simulink model "PID_Controller"  (R2020b)
settings: Solver=VariableStepAuto  StartTime=0.0  StopTime=1  FixedStep=Ts  RelTol=1e-3
model workspace (MAT data in the model file):
  Kd = Simulink.Parameter
  Kd.Value = 0.18
  Kd.DataType = 'auto'
  Kd.Dimensions = [1 1]
  Ki = Simulink.Parameter
  Ki.Value = 650.5
  Ki.DataType = 'auto'
  Ki.Dimensions = [1 1]
  Kp = Simulink.Parameter
  Kp.Value = 24.19
  Kp.DataType = 'auto'
  Kp.Dimensions = [1 1]
  N = Simulink.Parameter
  N.Value = 44124.63
  N.DataType = 'auto'
  N.Dimensions = [1 1]
  Ts = Simulink.Parameter
  Ts.Value = 0.01
  Ts.DataType = 'auto'
  Ts.Dimensions = [1 1]
settings Model: DataDictionary=motor1.sldd  Creator=Lenovo  LastModifiedBy=HP
settings DataIOCC: SaveOutput=off  SaveTime=off

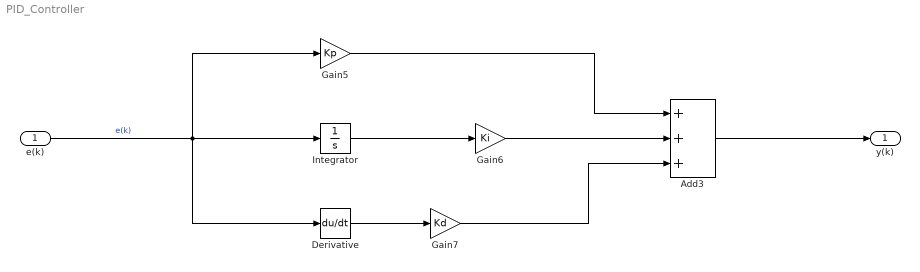
== system PID_Controller ==
  e(k) : Inport  OutDataTypeStr=double  PortDimensions=1  SampleTime=0
  Add3 : Sum  Inputs=+++
  Derivative : Derivative
  Gain5 : Gain  Gain=Kp
  Gain6 : Gain  Gain=Ki
  Gain7 : Gain  Gain=Kd
  Integrator : Integrator
  y(k) : Outport  OutDataTypeStr=double  PortDimensions=1  SampleTime=0
  wires:
  Gain5/1 -> Add3/1
  Add3/1 -> y(k)/1
  Gain7/1 -> Add3/3
  Gain6/1 -> Add3/2
  e(k)/1 -> Derivative/1, Integrator/1, Gain5/1  "e(k)"
  Integrator/1 -> Gain6/1
  Derivative/1 -> Gain7/1
